simulink model "tether000_thmc"  (R2022a)
settings: Solver=ode15s  StartTime=0.0  StopTime=simDuration  FixedStep=.1  RelTol=1e-3
values from neighbouring files (symbols this model uses):
  env = ENV.env    [tether000Test_ts.m]    (also in tether000_tsmc.m)
  tetherLengths = [200 200]    [tether000_tsmc.m]
libraries: tethers_cl x1
settings Model: Creator=James Reed  LastModifiedBy=lhill8
settings SolverCC: AlgebraicLoopSolver=TrustRegion
settings DebuggingCC: UnconnectedInputMsg=warning  UnconnectedOutputMsg=warning  UnconnectedLineMsg=warning  SFMachineParentedDataDiag=warning  ArithmeticOperatorsInVariantConditions=warning
settings SFSimCC: CustomCodeUndefinedFunction=UseInterfaceOnly

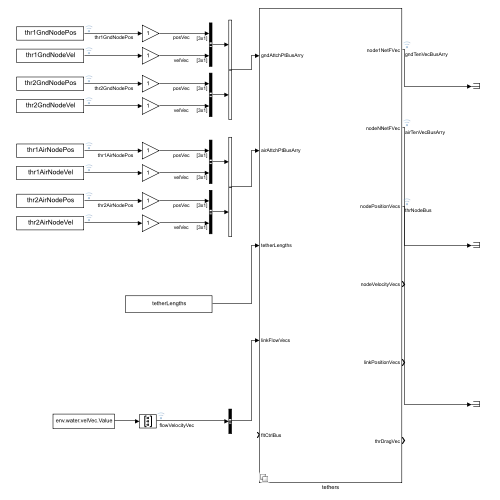
[thumbnail: Simulink's stored preview of the top-level diagram]
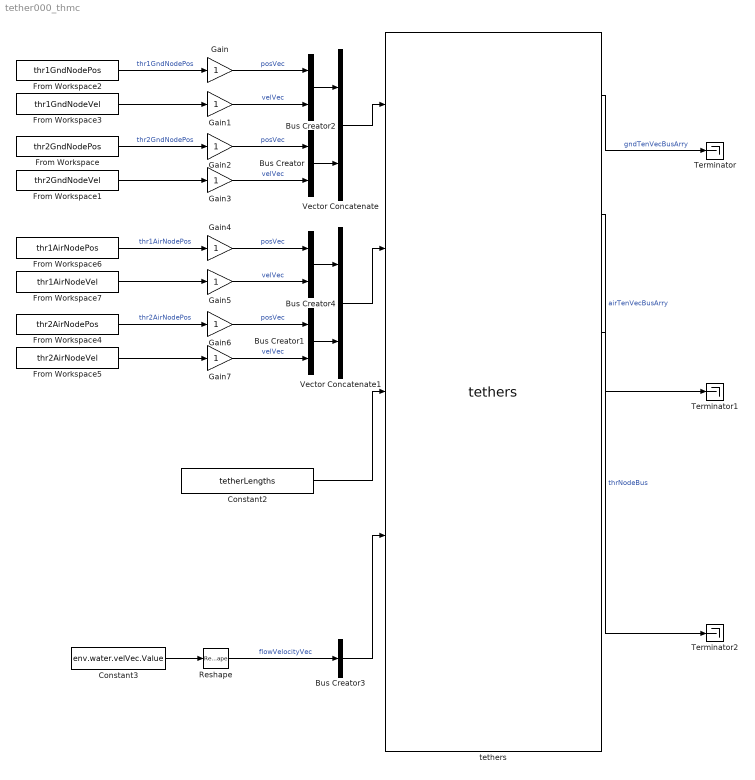
== system tether000_thmc ==
  Bus Creator{,1..2,4} (4 alike) : BusCreator  Inputs=2  OutDataTypeStr=Bus: thrAttachPtKinematicsBus  NonVirtualBus=on
  Bus Creator3 : BusCreator  Inputs=1  OutDataTypeStr=Bus:envBus
  Constant2 : Constant  Value=tetherLengths
  Constant3 : Constant  Value=env.water.velVec.Value
  From Workspace : FromWorkspace  VariableName=thr2GndNodePos
  From Workspace1 : FromWorkspace  VariableName=thr2GndNodeVel
  From Workspace2 : FromWorkspace  VariableName=thr1GndNodePos
  From Workspace3 : FromWorkspace  VariableName=thr1GndNodeVel
  From Workspace4 : FromWorkspace  VariableName=thr2AirNodePos
  From Workspace5 : FromWorkspace  VariableName=thr2AirNodeVel
  From Workspace6 : FromWorkspace  VariableName=thr1AirNodePos
  From Workspace7 : FromWorkspace  VariableName=thr1AirNodeVel
  Gain{,1..7} (8 alike) : Gain
  Reshape : Reshape  OutputDimensionality=Column vector (2-D)
  Terminator : Terminator
  Terminator1 : Terminator
  Terminator2 : Terminator
  Vector Concatenate : Concatenate
  Vector Concatenate1 : Concatenate
  tethers : tethers_cl/tethers  SystemSampleTime=-1  VariantActivationTime=update diagram  Latency=0  AutoFrameSizeCalculation=off
  wires:
  Constant2/1 -> tethers/3
  tethers/1 -> Terminator/1  "gndTenVecBusArry"
  From Workspace/1 -> Gain2/1  "thr2GndNodePos"
  From Workspace1/1 -> Gain3/1
  Constant3/1 -> Reshape/1
  Bus Creator3/1 -> tethers/4
  Reshape/1 -> Bus Creator3/1  "flowVelocityVec"
  From Workspace3/1 -> Gain1/1
  From Workspace2/1 -> Gain/1  "thr1GndNodePos"
  Bus Creator2/1 -> Vector Concatenate/1
  Bus Creator/1 -> Vector Concatenate/2
  Vector Concatenate/1 -> tethers/1
  Vector Concatenate1/1 -> tethers/2
  Bus Creator1/1 -> Vector Concatenate1/2
  Bus Creator4/1 -> Vector Concatenate1/1
  From Workspace6/1 -> Gain4/1  "thr1AirNodePos"
  From Workspace7/1 -> Gain5/1
  From Workspace5/1 -> Gain7/1
  From Workspace4/1 -> Gain6/1  "thr2AirNodePos"
  tethers/2 -> Terminator1/1  "airTenVecBusArry"
  tethers/3 -> Terminator2/1  "thrNodeBus"
  Gain/1 -> Bus Creator2/1  "posVec"
  Gain1/1 -> Bus Creator2/2  "velVec"
  Gain2/1 -> Bus Creator/1  "posVec"
  Gain3/1 -> Bus Creator/2  "velVec"
  Gain4/1 -> Bus Creator4/1  "posVec"
  Gain5/1 -> Bus Creator4/2  "velVec"
  Gain6/1 -> Bus Creator1/1  "posVec"
  Gain7/1 -> Bus Creator1/2  "velVec"
